simulink model "model2012b_mdl"  (Simulink 8.0)
settings: Solver=FixedStepDiscrete  StartTime=0.0  StopTime=100  FixedStep=0.1  RelTol=1e-3
values from neighbouring files (symbols this model uses):
  Li = a    [lab_script.m]
  Ts = 1    [lab_script.m]
libraries: commrandsrc2 x1, dspsrcs4 x1
settings Model: Creator=Ира  LastModifiedBy=Leonid
settings SolverCC: AutoInsertRateTranBlk=on
settings DataIOCC: SaveFormat=StructureWithTime  SignalLoggingSaveFormat=ModelDataLogs
settings OptimizationCC: ExpressionDepthLimit=128
settings DebuggingCC: UnderspecifiedInitializationDetection=Simplified  MergeDetectMultiDrivingBlocksExec=error  SolverPrmCheckMsg=none  FcnCallInpInsideContextMsg=EnableAllAsWarning  FrameProcessingCompatibilityMsg=error  StateNameClashWarn=none
settings HardwareCC: ProdIntDivRoundTo=Zero  ProdEndianess=LittleEndian  ProdHWDeviceType=Specified
settings CodeAppCC: CustomSymbolStrType=$N$R$M_T
settings GRTTargetCC: CodeReplacementLibrary=C89/C90 (ANSI)  CombineOutputUpdateFcns=off  GRTInterface=on

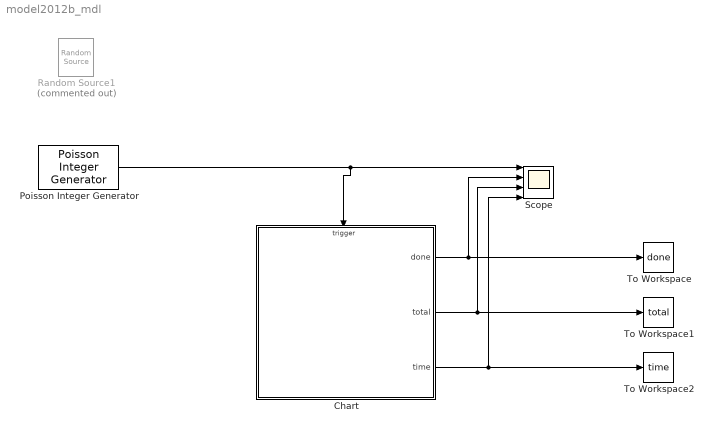
== system model2012b_mdl ==
  Chart : Stateflow chart  TreatAsAtomicUnit=on
      settings: PermitHierarchicalResolution=ParametersOnly
  Poisson Integer Generator : commrandsrc2/Poisson Integer Generator  lambda=1/Li  seed=0  Ts=Ts  sampPerFrame=1  outDataType=uint8
  Random Source1 : dspsrcs4/Random Source  Commented=on  SrcType=Gaussian  NormMethod=Sum of uniform values  CltLength=12  MinVal=0  MaxVal=1  MeanVal=Li  VarVal=1  RepMode=Repeatable  rawSeed=1  IsInherit=off  SampMode=Discrete  SampTime=Ts  SampFrame=1  DataType=Single  OutComplex=Real
  Scope : Scope  NumInputPorts=4
      settings: TimeRange=auto  MaxDataPoints=5000  SaveToWorkspace=off  SaveName=ScopeData  YMin=-4.47408~-11.875~-89.875~-1138.25  YMax=4.78891~106.875~808.875~10244.25  SampleTime=-1
  To Workspace : ToWorkspace  VariableName=done  SampleTime=Ts
  To Workspace1 : ToWorkspace  VariableName=total  SampleTime=Ts
  To Workspace2 : ToWorkspace  VariableName=time  SampleTime=Ts
  wires:
  Chart/1(done) -> To Workspace/1, Scope/2
  Chart/2(total) -> To Workspace1/1, Scope/3
  Chart/3(time) -> To Workspace2/1, Scope/4
  Poisson Integer Generator/1 -> Scope/1, Chart/Trigger

== stateflow chart Chart ==
  state Q1 [parallel]
    settings: executionOrder=2
    state ProcessQ1 [parallel]
      settings: executionOrder=1
      state free/
      state busy/
        entry:bt1=ml('prand(1/Lo)');
        to1=t;
        during: time++;
        exit: done++;
      Q1.ProcessQ1.free -> Q1.ProcessQ1.busy : setrequest
      (default) -> Q1.ProcessQ1.free
      (junction 37) -> Q1.ProcessQ1.free [order 2]
      (junction 37) -> Q1.ProcessQ1.busy [order 1] : [nq1>0]
          | {send(getrequest, QueueQ1);}
      Q1.ProcessQ1.busy -> (junction 37) : [t-to1>=bt1]
    state QueueQ1 [parallel]
      settings: executionOrder=2
      state empty/
      state stored/
        on setrequest: nq1++;
        on getrequest: nq1--;
        during:time=time+nq1;
      state full/
        during:time=time+nq1;
      Q1.QueueQ1.empty -> Q1.QueueQ1.stored : setrequest/
          | nq1++;
      (default) -> Q1.QueueQ1.empty
      Q1.QueueQ1.stored -> Q1.QueueQ1.empty [order 2] : [nq1==0]
      Q1.QueueQ1.full -> Q1.QueueQ1.stored : getrequest/
          | nq1--;
      Q1.QueueQ1.stored -> Q1.QueueQ1.full [order 1] : [nq1==ml.nqm1]
  state Q2 [parallel]
    settings: executionOrder=3
    state ProcessQ2 [parallel]
      settings: executionOrder=1
      state free/
      state busy/
        entry:bt2=ml('prand(1/Lo)');
        to2=t;
        during: time++;
        exit: done++;
      Q2.ProcessQ2.free -> Q2.ProcessQ2.busy : setrequest
      (default) -> Q2.ProcessQ2.free
      (junction 48) -> Q2.ProcessQ2.busy [order 1] : [nq2>0]
          | {send(getrequest, QueueQ2);}
      (junction 48) -> Q2.ProcessQ2.free [order 2]
      Q2.ProcessQ2.busy -> (junction 48) : [t-to2>=bt2]
    state QueueQ2 [parallel]
      settings: executionOrder=2
      state full/
        during:time=time+nq2;
      state stored/
        on setrequest: nq2++;
        on getrequest: nq2--;
        during:time=time+nq2;
      state empty/
      (default) -> Q2.QueueQ2.empty
      Q2.QueueQ2.empty -> Q2.QueueQ2.stored : setrequest/
          | nq2++;
      Q2.QueueQ2.stored -> Q2.QueueQ2.empty [order 2] : [nq2==0]
      Q2.QueueQ2.full -> Q2.QueueQ2.stored : getrequest/
          | nq2--;
      Q2.QueueQ2.stored -> Q2.QueueQ2.full [order 1] : [nq2==ml.nqm2]
  state Active [parallel]
    settings: executionOrder=1
    state main/
    (default) -> main
    (junction 21) -> (junction 22)
    main -> (junction 21) : request/
        | total++;
    (junction 22) -> Active [order 1] : [in(Q1.ProcessQ1.free)]
        | {send(setrequest, Q1.ProcessQ1)}
    (junction 25) -> main [order 2]
    (junction 22) -> (junction 23) [order 2]
    (junction 23) -> Active [order 1] : [in(Q2.ProcessQ2.free)]
        | {send(setrequest, Q2.ProcessQ2)}
    (junction 23) -> (junction 24) [order 2]
    (junction 24) -> Active [order 1] : [~in(Q1.QueueQ1.full)]
        | {send(setrequest, Q1.QueueQ1)}
    (junction 24) -> (junction 25) [order 2]
    (junction 25) -> Active [order 1] : [~in(Q2.QueueQ2.full)]
        | {send(setrequest, Q2.QueueQ2)}
  data: bt1 local double; to1 local double; nq1 local double; nq2 local double; to2 local double; bt2 local double; done output double; total output double; time output double
  data bt1 settings: description=% length of queue
  data to1 settings: description=% length of queue
  data nq1 settings: description=% length of queue
  data nq2 settings: description=% length of queue
  data to2 settings: description=% length of queue
  data bt2 settings: description=% length of queue
  data done settings: description=% length of queue
  data total settings: description=% length of queue
  data time settings: description=% length of queue
  events: request input RISING_EDGE_EVENT; setrequest local FUNCTION_CALL_EVENT; getrequest local FUNCTION_CALL_EVENT
